simulink model "pendulum"  (R2017b)
settings: Solver=ode4  StartTime=0.0  StopTime=10.0  FixedStep=0.0001  RelTol=1e-3
settings Model: Creator=lyx  LastModifiedBy=lyx

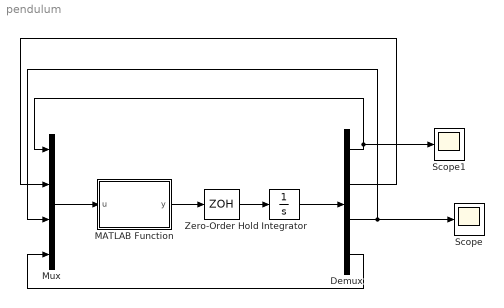
== system pendulum ==
  Demux : Demux
  Integrator : Integrator  InitialCondition=[0 0 3.14/18 0]
  MATLAB Function : MATLAB Function  TreatAsAtomicUnit=on
  Mux : Mux
  Scope : Scope
  Scope1 : Scope
  Zero-Order Hold : ZeroOrderHold  SampleTime=0.005
  wires:
  MATLAB Function/1(y) -> Zero-Order Hold/1
  Mux/1 -> MATLAB Function/1(u)
  Integrator/1 -> Demux/1
  Demux/1 -> Mux/1, Scope1/1
  Demux/2 -> Mux/2
  Demux/3 -> Scope/1, Mux/3
  Demux/4 -> Mux/4
  Zero-Order Hold/1 -> Integrator/1

== matlab function pendulum/MATLAB Function ==
  data: u input; y output
function y = fcn(u)
m = 0.109;
M = 0.01;
L = 0.25;
g = 9.8;
y = zeros(1,4);
x = u(1); x_dot = u(2); theta = u(3); theta_dot = u(4);



K = [-0.7071  -1.1183 -6.367 -1.0294];

c = -K*u;

y(1) = x_dot;
y(3) = theta_dot;

y(2) = (-m*g*cos(theta)*sin(theta) + theta_dot^2 *m *L * sin(theta) + c)/(M+m*sin(theta)^2);
y(4) = ((M+m) *g * sin(theta) - theta_dot^2*m*L*sin(theta)*cos(theta) - c*cos(theta));
y(4) = y(4) / (M+m*sin(theta)^2) /L;
